simulink model "SynchGenerator_DQ_ExciterAndTurbine"  (R2016b)
settings: Solver=FixedStepAuto  StartTime=0.0  StopTime=20  FixedStep=0.00005  MaxStep=200e-6  RelTol=1e-4  EnableMultiTasking=on
PreLoadFcn:
  | % Machine parameters from Kundur Examples 3.1, 3.2,  8.1 (pages 91,102, 345)
  | % "Power System Stability and Control"  McGraw-Hill  book, 1994
  | % --------------------------------------------------------------------
  | % Nominal parameters
  | Pn=  555e6;   % three-pahse nominal power (VA)
  | Vn=  24e3;    % nominal LL volatge (Vrms)
  | fn=  60;      % nominal frequency (Hz)
  | ifn= 1300;    % nominal field current (A)
  | % Note: ifn is deduced from stator-field mutual inductance Lsfd
  | %       Lsfd = Vn/sqrt(3)*sqrt(2)/ifn/wn
  | % ->     ifn = sqrt(2/3)*Vn/Lsfd/(2*pi*60)  = 1300 A
  | 
  | 
  | % Stator RL parameters (SI)
  | Rs= 0.0031;     % resistance (ohms)
  | Ll= 0.4129e-3;  % leakage inductance (H)
  | Lmd=4.5696e-3;  % d-axis magnetizing inductance (H)
  | Lmq=4.432e-3;   % q-axis magnetizing inductance (H)
  | 
  | % Field RL parameters (SI)
  | Rf= 0.0715;    %  resistance (ohms)
  | Lffd= 0.57692; %  self inductance (H)
  | % Note: Field leakage inductance Llfd wiil be later deduced from:
  | % Llfd_pu= Lffd_pu-Lmd_pu
  | 
  | % Damper RL parameters from Kundur Example 3.2
  | Rkd_pu   = 0.0284;
  | Llkd_pu  = 0.1713;
  | Rkq1_pu  = 0.00619;
  | Llkq1_pu = 0.7252;
  | Rkq2_pu  = 0.02368;
  | Llkq2_pu = 0.125;
  | 
  | % Stator base values
  | wbase=2*pi*fn;
  | Vsbase=Vn/sqrt(3)*sqrt(2);
  | Isbase=Pn/Vn/sqrt(3)*sqrt(2);
  | Zsbase=Vn^2/Pn;
  | Lsbase=Zsbase/wbase;
  | 
  | %Stator parameters in PU
  | Rs_pu=Rs/Zsbase;
  | Ll_pu=Ll/Lsbase;
  | Lmd_pu=Lmd/Lsbase;
  | Lmq_pu=Lmq/Lsbase;
  | 
  | % Field base values
  | Ifbase=ifn*Lmd_pu;
  | Vfbase=Pn/Ifbase;
  | Zfbase=Vfbase/Ifbase;
  | Lfbase=Zfbase/wbase;
  | 
  | % Transformation ratio Ns/Nf
  | Ns_Nf=2/3*Ifbase/Isbase;
  | 
  | % Field parameters in PU
  | Rf_pu=Rf/Zfbase;
  | Lffd_pu=Lffd/Lfbase;      % self inductance (pu)
  | Llfd_pu=Lffd_pu - Lmd_pu; % leakage inductance (pu)
  | Llfd= Llfd_pu*Lfbase;     % leakage inductance (H)
  | 
  | % Field parameters referred to the stator
  | Rf_prime=Rf*3/2*Ns_Nf^2;
  | Llfd_prime=Llfd*3/2*Ns_Nf^2;
  | 
  | % Nominal field voltage
  | Vfn=Rf*ifn;
  | % Nominal field voltage and current referred to stator
  | Vfn_prime=Rf_pu/Lmd_pu*Vsbase;
  | Ifn_prime=Isbase/Lmd_pu;
  | 
  | % Inertia
  | H= 3.7; % sec
  | wm= 2*pi*60; %rad/s
  | J= 2*H*Pn/wm^2; % kg.m^2
values from neighbouring files (symbols this model uses):
  Ef1 = 3.1    [param_Exciter_Eremia.m]
  Ef2 = 2.3    [param_Exciter_Eremia.m]
  Fa_t = 0.3    [param_Governor_Kundur.m]
  Fb_t = 0.3    [param_Governor_Kundur.m]
  Fc_t = 0.4    [param_Governor_Kundur.m]
  Ka_e = 46    [param_Exciter_Eremia.m]
  Ke_e = -0.043478260869565    (= -0.0434782608696)    [param_Exciter_Eremia.m]
  Kf_e = 0.1    [param_Exciter_Eremia.m]
  Kg_t = 20    [param_Governor_Kundur.m]
  Se_1 = 0.33    [param_Exciter_Eremia.m]
  Se_2 = 0.1    [param_Exciter_Eremia.m]
  Ta_e = 0.06    [param_Exciter_Eremia.m]
  Tb_t = 7    [param_Governor_Kundur.m]
  Te_e = 0.46    [param_Exciter_Eremia.m]
  Tf_e = 1    [param_Exciter_Eremia.m]
  Tsm_t = 0.3    [param_Governor_Kundur.m]
  Tsr_t = 0.1    [param_Governor_Kundur.m]
libraries: powerlib x10, sps_avr x1
Description:
  | Copyright 2008-2016 The MathWorks, Inc.
settings Model: Creator=MathWorks  LastModifiedBy=mmi-vsa
settings DataIOCC: Decimation=10  LimitDataPoints=on  SaveFormat=Array
settings OptimizationCC: ExpressionDepthLimit=2147483647  LifeSpan=inf
settings DebuggingCC: UnderspecifiedInitializationDetection=Classic  MergeDetectMultiDrivingBlocksExec=none  SolverPrmCheckMsg=warning  UnconnectedInputMsg=none  UnconnectedOutputMsg=none  UnconnectedLineMsg=none  StateNameClashWarn=warning  SFUnexpectedBacktrackingDiag=warning  SFNoUnconditionalDefaultTransitionDiag=warning  SFExecutionAtInitializationDiag=none
settings HardwareCC: ProdBitPerPointer=32  ProdBitPerSizeT=32  ProdBitPerPtrDiffT=32  ProdLargestAtomicFloat=None  ProdIntDivRoundTo=Undefined  ProdEndianess=Unspecified  ProdWordSize=32  ProdHWDeviceType=32-bit Generic
settings ModelReferenceCC: PropagateSignalLabelsOutOfModel=off
settings GRTTargetCC: TargetLangStandard=C89/C90 (ANSI)  GeneratePreprocessorConditionals=Disable all
settings ConfigComp: CovMetricSettings=dw  CovHtmlReporting=on  CovSaveCumulativeToWorkspaceVar=on  CovSaveSingleToWorkspaceVar=on  CovExternalEMLEnable=off  CovSFcnEnable=off

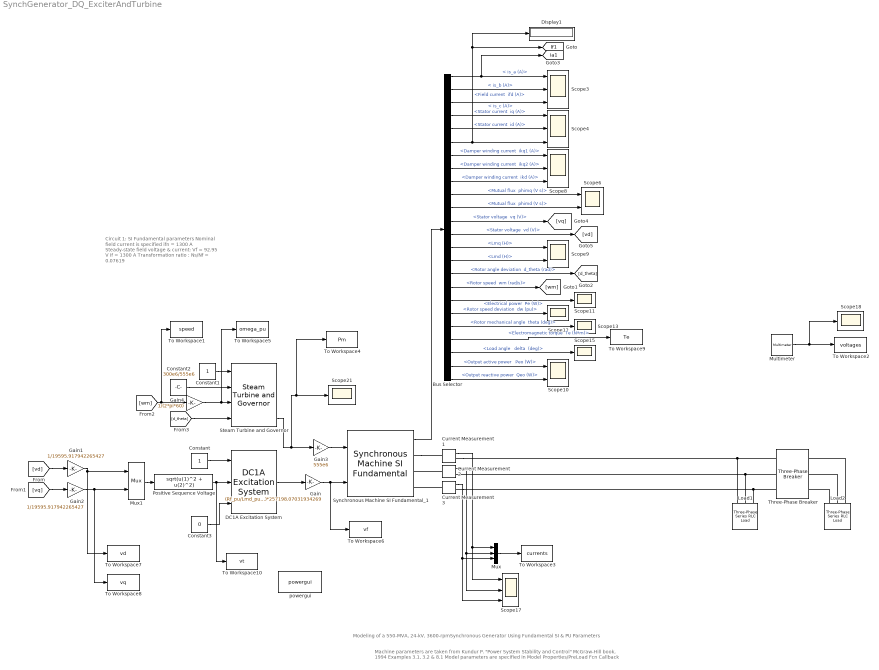
== system SynchGenerator_DQ_ExciterAndTurbine ==
  note: Circuit 1: SI Fundamental parameters
      |
      | Nominal field current is specified
      |      ifn = 1300 A
      | Steady-state field voltage & current:
      |     Vf = 92.95 V
      |     If  = 1300 A
      | Transformation ratio :
      |     Ns/Nf = 0.07619
  note: Machine parameters are taken from Kundur P.  "Power System Stability and Control" McGraw-Hill  book, 1994 Examples 3.1, 3.2 &  8.1
      | Model parameters are specified  in Model Properties/PreLoad Fcn Callback
  note: Modeling of a 550-MVA, 24-kV, 3600-rpmSynchronous Generator Using Fundamental SI & PU Parameters
  Bus Selector : BusSelector  OutputSignals="Stator current. is_a (A),Stator current. is_b (A),Stator current. is_c (A),dq0 components.Stator current  iq (A),dq0 components.Stator current  id (A),dq0 components.Field current  ifd (A),dq0 components.Damper winding current  ikq1 (A),dq0 components.Damper winding current  ikq2 (A),dq0 components.Damper winding current  ikd (A),dq0 components.Mutual flux  phimq (V s),dq0 components.Mutual flux  phimd (V s),dq0 components.Stator voltage  vq (V),dq0 components.Stator voltage  vd (V),dq0 components.Lmq (H),dq0 components.Lmd (H),Mechanical.Rotor angle deviation  d_theta (rad),Mechanical.Rotor speed  wm (rad/s),Mechanical.Electrical power  Pe (W),Mechanical.Rotor speed deviation  dw (pu),Mechanical.Rotor mechanical angle  theta (deg),Mechanical.Electromagnetic torque  Te (N*m),Load angle   delta  (deg),Output active power   Peo (W),Output reactive power  Qeo (W)"
  Constant : Constant
  Constant1 : Constant
  Constant2 : Constant  Value=300e6/555e6
  Constant3 : Constant  Value=0
  Current Measurement1 : powerlib/Measurements/Current Measurement  PhasorSimulation=off  OutputType=Complex  PSBequivalent=0
  Current Measurement2 : powerlib/Measurements/Current Measurement  PhasorSimulation=off  OutputType=Complex  PSBequivalent=0
  Current Measurement3 : powerlib/Measurements/Current Measurement  PhasorSimulation=off  OutputType=Complex  PSBequivalent=0
  DC1A Excitation System : sps_avr/DC1A Excitation System  Tr=Tr_e  KaTa=[Ka_e Ta_e]  VRminmax=[-0.9 1.0]  KfTf=[Kf_e Tf_e]  TbTc=[0 0]  KeTe=[Ke_e Te_e]  Efd12=[Ef1 Ef2]  SeEfd12=[Se_1 Se_2]  v0=[1 1]  TsBlock=0
  Display1 : Display
  Gain : Gain  Gain=(Rf_pu/Lmd_pu)*257198.07031934269
  Gain1 : Gain  Gain=1/19595.917942265427
  Gain2 : Gain  Gain=1/19595.917942265427
  Gain3 : Gain  Gain=555e6
  Gain4 : Gain  Gain=1/(2*pi*60)
  Load1 : powerlib/Elements/Three-Phase Series RLC Load  LConnTagsString=A|B|C  Configuration=Y (grounded)  NominalVoltage=24e3  Vabc=[1e3 1e3 1e3]  Vabcp=[1e3 1e3 1e3]  NominalFrequency=60  UnbalancedPower=off  ActivePower=300e6  InductivePower=0  CapacitivePower=0  Pabc=[10e3 9e3 11e3]  QLabc=[100 90 110]  QCabc=[100 90 110]  Pabcp=[10e3 9e3 11e3]  QLabcp=[100 90 110]  QCabcp=[100 90 110]  Measurements=Branch voltages and currents  LoadType=constant Z
  Load2 : powerlib/Elements/Three-Phase Series RLC Load  LConnTagsString=A|B|C  Configuration=Y (grounded)  NominalVoltage=24e3  Vabc=[1e3 1e3 1e3]  Vabcp=[1e3 1e3 1e3]  NominalFrequency=60  UnbalancedPower=off  ActivePower=30e6  InductivePower=0  CapacitivePower=0  Pabc=[10e3 9e3 11e3]  QLabc=[100 90 110]  QCabc=[100 90 110]  Pabcp=[10e3 9e3 11e3]  QLabcp=[100 90 110]  QCabcp=[100 90 110]  Measurements=Branch voltages and currents  LoadType=constant Z
  Multimeter : powerlib/Measurements/Multimeter  PhasorSimulation=off  OutputType=Complex  sel=[1 2 3]  L=12  Gain=[1 1 1]  yselected={'Uag: Load1','Ubg: Load1','Ucg: Load1'};  PSBOutputType=1  PSBequivalent=0  AxesSetting=[0,0.1,-100,100]  Display=0  SavedBlockNames=-11
  Mux : Mux  Inputs=3
  Mux1 : Mux  Inputs=2
  Positive Sequence Voltage : Fcn  Expr=sqrt(u(1)^2 + u(2)^2)
  Scope10 : Scope  NumInputPorts=2
  Scope{11..13,15,18,21} (6 alike) : Scope
  Scope{3..4,8,17} (4 alike) : Scope  NumInputPorts=3
  Scope6 : Scope  NumInputPorts=2
  Scope9 : Scope  NumInputPorts=2
  Steam Turbine and Governor : powerlib/Machines/Steam Turbine and Governor  gentype=Tandem-compound (single mass)  reg1=[ 1 1/Kg_t 0 ]  reg2="[ Tsr_t  Tsm_t ]"  reg3=[-1 0.1 0 1]  N=3600  turb1="[ 0  0   Tb_t   0 ]"  turb2="[ Fc_t  0   Fb_t  Fa_t ]"  HA="[  1.5498   0.24894  0  0 ]"  KA="[  83.47  42.702  0  0 ]"  DA="[  0.3104  0.05  0  0 ]*8"  ini1=300e6/555e6  ini2=[2.7247e-008,-120.13]
  Synchronous Machine SI Fundamental_1 : powerlib/Machines/Synchronous Machine SI Fundamental  PresetModel=No  MechanicalLoad=Mechanical power Pm  ShowDetailedParameters=on  RotorType=Salient-pole  Units=SI fundamental parameters  MeasurementBus=off  NominalParameters="[ Pn  Vn    fn  ifn ]"  Stator="[ Rs    Ll    Lmd     Lmq ]"  Field="[Rf   Llfd ]*3/2*(Ns_Nf)^2"  Dampers2="[Rkd_pu Llkd_pu  Rkq1_pu  Llkq1_pu Rkq2_pu  Llkq2_pu ] .*[Zsbase  Lsbase  Zsbase  Lsbase  Zsbase  Lsbase]"  Dampers1="[Rkd_pu  Llkd_pu  Rkq1_pu  Llkq1_pu].*[Zsbase  Lsbase  Zsbase  Lsbase]"  Mechanical="[ J  0 1 ]"  PolePairs=1  InitialConditions=[0 -46.4745 10206.21 10206.21 10206.21 -180 -60 60 130.16]  SetSaturation=off  Saturation=[695.64,774.7,917.5,1001.6,1082.2,1175.9,1293.6,1430.2,1583.7;9660,10623,12243,13063,13757,14437,15180,15890,16567]  DisplayVfd=off  LoadFlowParameters=[2 0 0 0 0]  TsPowergui=0  TsBlock=-1  IterativeModel=Trapezoidal iterative (alg. loop)  IterativeDiscreteModel=Trapezoidal non iterative  BusType=swing  Pref=0  Qref=0  Qmin=-inf  Qmax=inf  PLF=0  QLF=0
  Three-Phase Breaker : powerlib/Elements/Three-Phase Breaker  InitialState=open  SwitchA=on  SwitchB=on  SwitchC=on  SwitchTimes=[0.1]  External=off  BreakerResistance=0.001  SnubberResistance=inf  SnubberCapacitance=0  Measurements=None
  To Workspace1 : ToWorkspace  VariableName=speed  SampleTime=-1
  To Workspace10 : ToWorkspace  VariableName=vt  SampleTime=-1
  To Workspace2 : ToWorkspace  VariableName=voltages  SampleTime=-1
  To Workspace3 : ToWorkspace  VariableName=currents  SampleTime=-1
  To Workspace4 : ToWorkspace  VariableName=Pm  SampleTime=-1
  To Workspace5 : ToWorkspace  VariableName=omega_pu  SampleTime=-1
  To Workspace6 : ToWorkspace  VariableName=vf  SampleTime=-1
  To Workspace7 : ToWorkspace  VariableName=vd  SampleTime=-1
  To Workspace8 : ToWorkspace  VariableName=vq  SampleTime=-1
  To Workspace9 : ToWorkspace  VariableName=Te  SampleTime=-1
  powergui : powerlib/powergui  Priority=1  SimulationMode=Discrete  SolverType=Backward Euler  SampleTime=5e-5  frequency=60  SPID=on  DisableSnubberDevices=on  DisableRonSwitches=off  DisableVfSwitches=off  SwTol=0  DisplayEquations=off  Interpol=off  ExternalGateDelay=off  methode=off  Ts=0  FunctionMessages=off  echomessages=off  HookPort=off  EnableUseOfTLC=off  x0status=blocks  frequencyindice=60  Pbase=100e6  ErrMax=0.0001  Iterations=50  UnitsV=kV  UnitsW=MW  buscounter=0  RestoreLinks=warning  ResistiveCurrentMeasurement=off  Frange=[0:2:500]  Ylog=off  Xlog=on  ShowGrid=off  save=off  variable=ZData  structure=0  ZoomFFT=off  StartTime=0.0  cycles=1  DisplayStyle=1  fundamental=60  FreqAxis=off  MaxFrequency=1000  frequencyindicesteady=1  RmsSteady=1  display=off
  tag scope: If1=global, ia1=global
  wires:
  Synchronous Machine SI Fundamental_1/1 -> Bus Selector/1
  Bus Selector/6 -> Scope4/3, Display1/1, [If1]  "<Field current  ifd (A)>"
  Bus Selector/1 -> [ia1], Scope3/1  "< is_a (A)>"
  Bus Selector/2 -> Scope3/2  "< is_b (A)>"
  Bus Selector/3 -> Scope3/3  "< is_c (A)>"
  Bus Selector/4 -> Scope4/1  "<Stator current  iq (A)>"
  Bus Selector/5 -> Scope4/2  "<Stator current  id (A)>"
  Bus Selector/10 -> Scope6/1  "<Mutual flux  phimq (V s)>"
  Bus Selector/11 -> Scope6/2  "<Mutual flux  phimd (V s)>"
  Bus Selector/12 -> [vq]  "<Stator voltage  vq (V)>"
  Bus Selector/13 -> [vd]  "<Stator voltage  vd (V)>"
  Bus Selector/7 -> Scope8/1  "<Damper winding current  ikq1 (A)>"
  Bus Selector/8 -> Scope8/2  "<Damper winding current  ikq2 (A)>"
  Bus Selector/9 -> Scope8/3  "<Damper winding current  ikd (A)>"
  Bus Selector/14 -> Scope9/1  "<Lmq (H)>"
  Bus Selector/15 -> Scope9/2  "<Lmd (H)>"
  Bus Selector/16 -> [d_theta]  "<Rotor angle deviation  d_theta (rad)>"
  Bus Selector/17 -> [wm]  "<Rotor speed  wm (rad/s)>"
  Bus Selector/18 -> Scope11/1  "<Electrical power  Pe (W)>"
  Bus Selector/19 -> Scope12/1  "<Rotor speed deviation  dw (pu)>"
  Bus Selector/20 -> Scope13/1  "<Rotor mechanical angle  theta (deg)>"
  Bus Selector/21 -> To Workspace9/1  "<Electromagnetic torque  Te (N*m)>"
  Bus Selector/22 -> Scope15/1  "<Load angle   delta  (deg)>"
  Bus Selector/23 -> Scope10/1  "<Output active power   Peo (W)>"
  Bus Selector/24 -> Scope10/2  "<Output reactive power  Qeo (W)>"
  Multimeter/1 -> Scope18/1, To Workspace2/1
  Mux/1 -> To Workspace3/1
  Current Measurement1/1 -> Scope17/1, Mux/1
  Current Measurement2/1 -> Scope17/2, Mux/2
  Current Measurement3/1 -> Scope17/3, Mux/3
  Gain3/1 -> Synchronous Machine SI Fundamental_1/1
  Gain/1 -> To Workspace6/1, Synchronous Machine SI Fundamental_1/2
  DC1A Excitation System/1 -> Gain/1
  [vd] -> Gain1/1
  [vq] -> Gain2/1
  Gain1/1 -> Mux1/1, To Workspace7/1
  Constant1/1 -> Steam Turbine and Governor/1
  Constant2/1 -> Steam Turbine and Governor/2
  [d_theta] -> Steam Turbine and Governor/4
  [wm] -> To Workspace1/1, Gain4/1
  Gain4/1 -> To Workspace5/1, Steam Turbine and Governor/3
  Steam Turbine and Governor/4 -> To Workspace4/1, Scope21/1, Gain3/1
  Gain2/1 -> Mux1/2, To Workspace8/1
  Mux1/1 -> Positive Sequence Voltage/1
  Positive Sequence Voltage/1 -> DC1A Excitation System/2, To Workspace10/1
  Constant/1 -> DC1A Excitation System/1
  Constant3/1 -> DC1A Excitation System/3
  connections:
  Synchronous Machine SI Fundamental_1/RConn1 -- Current Measurement1/LConn1
  Current Measurement2/LConn1 -- Synchronous Machine SI Fundamental_1/RConn2
  Current Measurement3/LConn1 -- Synchronous Machine SI Fundamental_1/RConn3
  Load2/LConn1 -- Three-Phase Breaker/RConn3
  Load2/LConn2 -- Three-Phase Breaker/RConn2
  Load2/LConn3 -- Three-Phase Breaker/RConn1
  Three-Phase Breaker/LConn3 -- Current Measurement3/RConn1 -- Load1/LConn3
  Three-Phase Breaker/LConn2 -- Current Measurement2/RConn1 -- Load1/LConn2
  Three-Phase Breaker/LConn1 -- Current Measurement1/RConn1 -- Load1/LConn1
